simulink model "testbench_sensor_distance"  (R2016b)
settings: Solver=FixedStepAuto  StartTime=0.0  StopTime=inf  RelTol=1e-3  EnableMultiTasking=on
libraries: legoev3lib x4
settings Model: SimulationMode=external  ExtModeTrigDuration=2  Creator=Shobhit  LastModifiedBy=karanverma
settings SolverCC: PositivePriorityOrder=on
settings OptimizationCC: LifeSpan=1  MaxStackSize=64
settings DebuggingCC: SFUnexpectedBacktrackingDiag=warning  SFNoUnconditionalDefaultTransitionDiag=warning  SFExecutionAtInitializationDiag=none
settings HardwareCC: ProdBitPerPointer=32  ProdBitPerSizeT=32  ProdBitPerPtrDiffT=32  ProdLargestAtomicInteger=Long  ProdWordSize=32  ProdHWDeviceType=ARM Compatible->ARM 9  UseEmbeddedCoderFeatures=off  UseSimulinkCoderFeatures=off
settings RTWCC: SystemTargetFile=ert.tlc  HardwareBoard=LEGO MINDSTORMS EV3  TLCOptions=-aInlineSetEventsForThisBaseRateFcn=TLC_FALSE -aSuppressMultiTaskScheduler=TLC_FALSE -aRateBasedStepFcn=0  TemplateMakefile=ert_default_tmf  Description=Embedded Coder  GenerateReport=on  Toolchain=Sourcery G++ Lite v2009q3  LaunchReport=on
settings CodeAppCC: ForceParamTrailComments=on  OperatorAnnotations=on  MATLABSourceComments=on
settings ERTTargetCC: ERTCustomFileBanners=off  SupportContinuousTime=on  SupportNonInlinedSFcns=on  SupportVariableSizeSignals=on  ModelStepFunctionPrototypeControlCompliant=off
settings ConfigComp: CovMetricSettings=dw  CovHtmlReporting=on  CovSaveCumulativeToWorkspaceVar=on  CovSaveSingleToWorkspaceVar=on  CovExternalEMLEnable=off

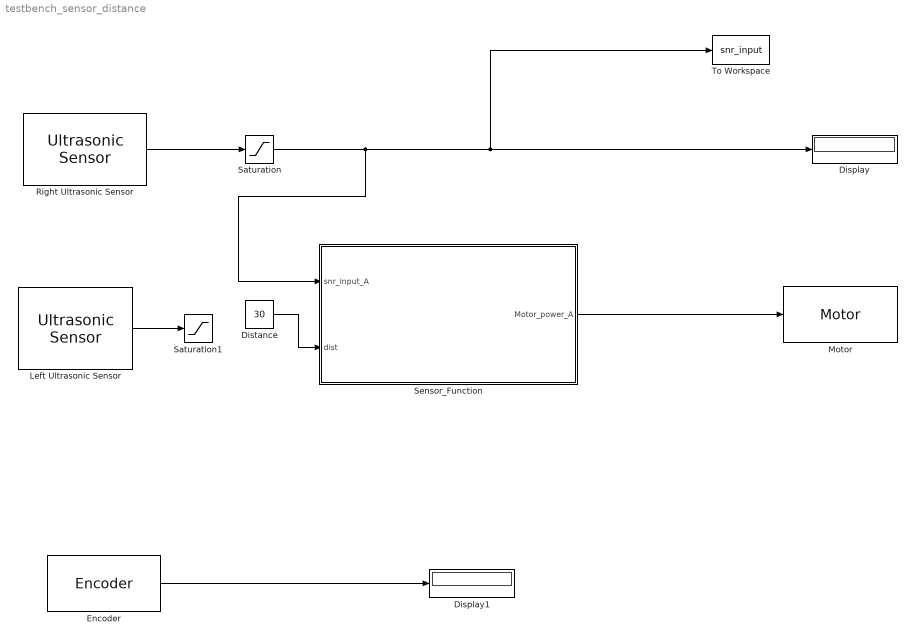
== system testbench_sensor_distance ==
  Display : Display
      settings: Format=decimal (Stored Integer)
  Display1 : Display
      settings: Format=decimal (Stored Integer)
  Distance : Constant  Value=30
  Encoder : legoev3lib/Encoder  portNumber=A  opMode=Reset by external signal  sampleTime=0.1
  Left Ultrasonic Sensor : legoev3lib/Ultrasonic Sensor  PortNumber=1  sampleTime=0.1
  Motor : legoev3lib/Motor  sportNumber=A  sstopAction=Brake
  Right Ultrasonic Sensor : legoev3lib/Ultrasonic Sensor  PortNumber=2  sampleTime=0.05
  Saturation : Saturate  UpperLimit=100  LowerLimit=3
  Saturation1 : Saturate  UpperLimit=100  LowerLimit=3
  Sensor_Function : MATLAB Function  TreatAsAtomicUnit=on
  To Workspace : ToWorkspace  VariableName=snr_input  SampleTime=-1
  wires:
  Sensor_Function/1(Motor_power_A) -> Motor/1
  Right Ultrasonic Sensor/1 -> Saturation/1
  Left Ultrasonic Sensor/1 -> Saturation1/1
  Saturation/1 -> To Workspace/1, Display/1, Sensor_Function/1(snr_input_A)
  Distance/1 -> Sensor_Function/2(dist)
  Encoder/1 -> Display1/1

== matlab function testbench_sensor_distance/Sensor_Function ==
  data: snr_input_A input; dist input; Motor_power_A output
function Motor_power_A  = fcn(snr_input_A,dist)
%#codegen
while 1
   if (snr_input_A<=dist)
      Motor_power_A=100;
   else
      Motor_power_A=0;
   end
   break;
end
% pause(10);
% while 1 
%     if (encA<=850)
%         Motor_power_A=50;
%     else
%         Motor_power_A=0;
%     end
%     break;
end
